simulink subsystem "HighLevelControlSUB"  (R2023a)
settings: Solver=VariableStepAuto  StartTime=0.0  StopTime=10.0  RelTol=1e-3
settings Model: Creator=romav  LastModifiedBy=romav

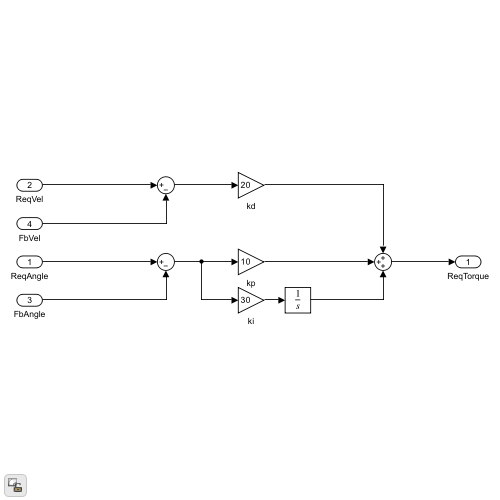
[thumbnail: Simulink's stored preview of the top-level diagram]
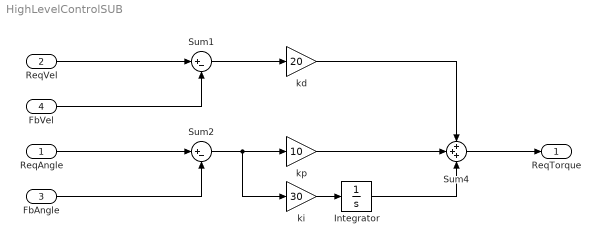
== system HighLevelControlSUB ==
  ReqAngle : Inport
  ReqVel : Inport  Port=2
  FbAngle : Inport  Port=3
  FbVel : Inport  Port=4
  Integrator : Integrator
  Sum1 : Sum  Inputs=|+-
  Sum2 : Sum  Inputs=|+-
  Sum4 : Sum  Inputs=+++
  kd : Gain  Gain=20
  ki : Gain  Gain=30
  kp : Gain  Gain=10
  ReqTorque : Outport
  wires:
  Integrator/1 -> Sum4/3
  FbVel/1 -> Sum1/2
  Sum2/1 -> kp/1, ki/1
  ReqAngle/1 -> Sum2/1
  ki/1 -> Integrator/1
  kd/1 -> Sum4/1
  FbAngle/1 -> Sum2/2
  kp/1 -> Sum4/2
  Sum4/1 -> ReqTorque/1
  ReqVel/1 -> Sum1/1
  Sum1/1 -> kd/1
